simulink model "SignalGen_rx"  (R2016a)
settings: Solver=FixedStepDiscrete  StartTime=0.0  StopTime=0.0333333  RelTol=1e-3
InitFcn:
  | SignalGen_Settings
values from neighbouring files (symbols this model uses):
  A = A(1:L/2+1)    [fft_analisys.m]
  DAC1 = ceil( DAC1_A  * PWM_Counter *             ( DAC1_H1 + DAC1_H2 + DAC1_H3) +               PWM_Offset )    [SignalGen_Pkg_Test.m]    (also in SignalGen_Settings.m)
  DAC2 = ceil( DAC2_A  * PWM_Counter *             ( DAC2_H1 + DAC2_H2 + DAC2_H3 + DAC2_H3) +               PWM_Offset )    [SignalGen_Pkg_Test.m]    (also in SignalGen_Settings.m)
  DAC3 = ceil( DAC3_A  * PWM_Counter *               DAC3_H1 +               PWM_Offset )    [SignalGen_Pkg_Test.m]    (also in SignalGen_Settings.m)
  DAC4 = ceil( DAC4_A  * PWM_Counter *             ( DAC4_H1 + DAC4_noise ) +               PWM_Offset )    [SignalGen_Pkg_Test.m]    (also in SignalGen_Settings.m)
  PWM_Max_Voltage = 3.3    [SignalGen_Pkg_Test.m]    (also in SignalGen_Settings.m)
  PWM_Offset = PWM_Counter/2    (= 180)    [SignalGen_Pkg_Test.m]    (also in SignalGen_Settings.m)
  PWM_Scale = PWM_Max_Voltage/PWM_Counter    (= 0.00916666666667)    [SignalGen_Pkg_Test.m]    (also in SignalGen_Settings.m)
  SampleNumber = 256    [SignalGen_Pkg_Test.m]    (also in SignalGen_Settings.m = 512)
undefined symbols (not defined in the file or in its folder): GPTRIP1SEL, GPTRIP2SEL, TZ1, TZ2
libraries: dspstat3 x4, c2802xlib x2, c280xlib x1, simulink x1
settings Model: ExtModeTrigDuration=8  Creator=Júlio Santos  LastModifiedBy=skelter_win
settings OptimizationCC: DefaultUnderspecifiedDataType=single  OptimizeModelRefInitCode=on  LifeSpan=1  MaxStackSize=512
settings HardwareCC: ProdBitPerChar=16  ProdBitPerInt=16  ProdBitPerPointer=32  ProdLargestAtomicInteger=Integer  ProdLargestAtomicFloat=None  ProdWordSize=16  ProdLongLongMode=on  ProdHWDeviceType=Texas Instruments->C2000
settings RTWCC: SystemTargetFile=ert.tlc  HardwareBoard=TI Piccolo F2806x  TemplateMakefile=ert_default_tmf  GenerateReport=on  Toolchain=Texas Instruments Code Composer Studio v6 (C2000)  BuildConfiguration=Faster Runs  IncludeHyperlinkInReport=on  LaunchReport=on  GenerateTraceInfo=on  GenerateTraceReport=on  GenerateTraceReportSl=on  GenerateTraceReportSf=on  GenerateTraceReportEml=on
settings CodeAppCC: ForceParamTrailComments=on  IgnoreCustomStorageClasses=off  OperatorAnnotations=on  SimulinkDataObjDesc=on  SFDataObjDesc=on  MATLABFcnDesc=on  InsertBlockDesc=on  MATLABSourceComments=on
settings ERTTargetCC: CodeReplacementLibrary=TI C28x  MemSecPackage=Simulink

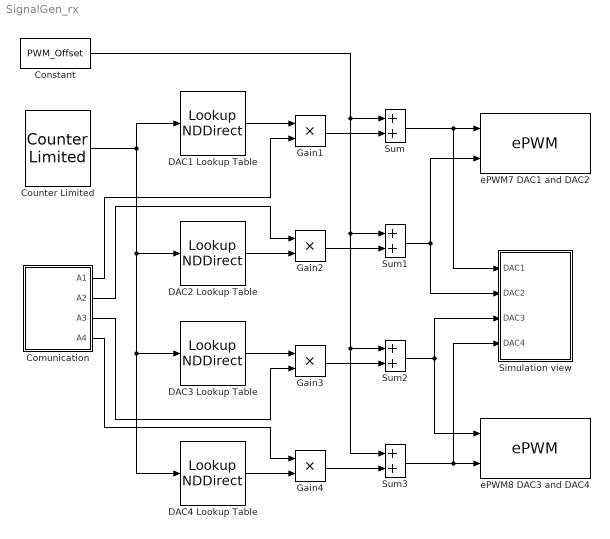
== system SignalGen_rx ==
  Comunication : Subsystem
  Constant : Constant  Value=PWM_Offset
  Counter Limited : simulink/Sources/Counter Limited  uplimit=SampleNumber-1  tsamp=SampleTime
  DAC1 Lookup Table : LookupNDDirect  NumberOfTableDimensions=1  Table=DAC1-PWM_Offset
  DAC2 Lookup Table : LookupNDDirect  NumberOfTableDimensions=1  Table=DAC2-PWM_Offset
  "DAC3 Lookup Table " : LookupNDDirect  NumberOfTableDimensions=1  Table=DAC3-PWM_Offset
  DAC4 Lookup Table : LookupNDDirect  NumberOfTableDimensions=1  Table=DAC4-PWM_Offset
  Gain{1..4} (4 alike) : Product
  Simulation view : Subsystem
  Sum{,1..3} (4 alike) : Sum  OutDataTypeStr=uint16
  ePWM7 DAC1 and DAC2 : c2802xlib/ePWM  useModule=ePWM7  ePWMxLINKTBPRD=Not Linked  periodUnits=Clock cycles  timerSource=Specify via dialog  timerPeriod_clk=PWM_Counter  timerPeriod_sec=2250  tbshadow=Counter equals to zero  countingMode=Up  phaseActiveEnable=Disable  phaseDirection=Count down after sync  phaseActive=0  synchronizationEnable=off  dcaevt1Sync=off  dcbevt1Sync=off  synchronizationOption=Disable  clockPrescale=1  HSclockPrescale=1  enswap=off  ePWMxAStatus=on  ePWMxAactionLogic1=Set  ePWMxAactionLogic2=Clear  ePWMxAactionLogic3=Clear  ePWMxAactionLogic4=Set  ePWMxAactionLogic5=Do nothing  ePWMxAactionLogic6=Do nothing  ePWMxALoadMode=Load on counter equals to zero (CTR=Zero)  ePWMxACSFenable=off  ePWMxACSFvalue=Forcing disable  ePWMxASFreload=Zero  ePWMxBStatus=on  ePWMxBactionLogic1=Set  ePWMxBactionLogic2=Clear  ePWMxBactionLogic3=Do nothing  ePWMxBactionLogic4=Do nothing  ePWMxBactionLogic5=Clear  ePWMxBactionLogic6=Set  ePWMxBLoadMode=Load on counter equals to zero (CTR=Zero)  ePWMxBCSFenable=off  ePWMxBCSFvalue=Forcing disable  ePWMxBSFreload=Zero  ePWNxBOutWay=off  ePWMxLINKCMPA=Not Linked  CMPAUnits=Clock cycles  CMPASource=Input port  CMPAValue_per=50  CMPAValue_clk=PWM_Offset  enCMPAshadow=Counter equals to zero  ePWMxLINKCMPB=Not Linked  CMPBUnits=Clock cycles  CMPBSource=Input port  CMPBValue_per=50  CMPBValue_clk=PWM_Offset  enCMPBshadow=Counter equals to zero  ePWMxLINKCMPC=Not Linked  CMPCUnits=Clock cycles  CMPCSource=Specify via dialog  CMPCValue_per=50  CMPCValue_clk=32000  enCMPCshadow=Counter equals to zero  ePWMxLINKCMPD=Not Linked  CMPDUnits=Clock cycles  CMPDSource=Specify via dialog  CMPDValue_per=50  CMPDValue_clk=32000  enCMPDshadow=Counter equals to zero  enableDBePWMxA=off  enableDBePWMxB=off  enhalfcycle=off  DBpolarity=Active high (AH)  DBedgeDelay=Positive  DBSource_ePWMxA=ePWMxA  DBSource_ePWMxB=ePWMxA  DBperiodSource=Specify via dialog  REDperiod=0  FEDperiod=0  adcstartModuleA=off  adcrequestEventA=First event  adcstartEventA=Digital Compare Module A Event 1 start of conversion (DCAEVT1.soc)  adcstartEventA_type2=Digital Compare Module A Event 1 start of conversion (DCAEVT1.soc)  adcstartModuleB=off  adcrequestEventB=First event  adcstartEventB=Counter equals to zero (CTR=Zero)  adcstartEventB_type2=Counter equals to zero (CTR=Zero)  intEn=off  intPrd=First event  intSel=Counter equals to zero (CTR=Zero)  intSel_type2=Counter equals to zero (CTR=Zero)  hrpe=off  enHRPWM=off  HRPWM_LoadMode=Counter equals to period (CTR=PRD)  HRPWM_CTLMode=Duty or Period control mode  HRPWM_EDGMode=Both edge  hrpeb=off  enHRPWMB=off  HRPWM_LoadModeB=Counter equals to zero (CTR=ZERO)  HRPWM_CTLModeB=Duty or Period control mode  HRPWM_EDGModeB=Both edge  enSFO=on  enautoconv=on  chopperEnable=off  chopperFrequency=1  chopperFirstwidth=1  chopperDuty=12.5%  tripZonesource=Specify via dialog  tzselOSHT1=off  tzselOSHT2=off  tzselOSHT3=off  tzselOSHDCAEV1=off  tzselOSHDCBEV1=off  tzselCBC1=off  tzselCBC2=off  tzselCBC3=off  tzselCBCDCAEV2=off  tzselCBCDCBEV2=off  tzselOSHT4=off  tzselOSHT5=off  tzselOSHT6=off  tzselCBC4=off  tzselCBC5=off  tzselCBC6=off  enTzOstIntr=off  enTzCbcIntr=off  enTzDCAEVT1Intr=off  enTzDCAEVT2Intr=off  enTzDCBEVT1Intr=off  enTzDCBEVT2Intr=off  ePWMxAforced=No action  ePWMxBforced=No action  DCAEVT1forced=No action  DCBEVT1forced=No action  DCAEVT2forced=No action  DCBEVT2forced=No action  dcah=Trip Zone 1 input (TZ1)  dcal=Trip Zone 2 input (TZ2)  dcbh=Trip Zone 1 input (TZ1)  dcbl=Trip Zone 2 input (TZ2)  dcah_type2=GPTRIP1SEL/(TZ1)  dcal_type2=GPTRIP2SEL/(TZ2)  dcbh_type2=GPTRIP1SEL/(TZ1)  dcbl_type2=GPTRIP2SEL/(TZ2)  gendcaevt1=Event disabled  gendcaevt2=Event disabled  gendcbevt1=Event disabled  gendcbevt2=Event disabled  dcaevt1src=DCAEVT1 with sync  dcaevt2src=DCAEVT2 with sync  dcbevt1src=DCBEVT1 with sync  dcbevt2src=DCBEVT2 with sync  pulsesel=Counter equals to zero (CTR=Zero)  blankinv=off  blankoffset=0  blankwidth=0  evsrcsel=Filtered version of DCAEVT1 (DCAEVT1FILT)  encape=off  PwmType=C2000
  ePWM8 DAC3 and DAC4 : c2802xlib/ePWM  useModule=ePWM8  ePWMxLINKTBPRD=Not Linked  periodUnits=Clock cycles  timerSource=Specify via dialog  timerPeriod_clk=PWM_Counter  timerPeriod_sec=2250  tbshadow=Counter equals to zero  countingMode=Up  phaseActiveEnable=Disable  phaseDirection=Count down after sync  phaseActive=0  synchronizationEnable=off  dcaevt1Sync=off  dcbevt1Sync=off  synchronizationOption=Disable  clockPrescale=1  HSclockPrescale=1  enswap=off  ePWMxAStatus=on  ePWMxAactionLogic1=Set  ePWMxAactionLogic2=Clear  ePWMxAactionLogic3=Clear  ePWMxAactionLogic4=Set  ePWMxAactionLogic5=Do nothing  ePWMxAactionLogic6=Do nothing  ePWMxALoadMode=Load on counter equals to zero (CTR=Zero)  ePWMxACSFenable=off  ePWMxACSFvalue=Forcing disable  ePWMxASFreload=Zero  ePWMxBStatus=on  ePWMxBactionLogic1=Set  ePWMxBactionLogic2=Clear  ePWMxBactionLogic3=Do nothing  ePWMxBactionLogic4=Do nothing  ePWMxBactionLogic5=Clear  ePWMxBactionLogic6=Set  ePWMxBLoadMode=Load on counter equals to zero (CTR=Zero)  ePWMxBCSFenable=off  ePWMxBCSFvalue=Forcing disable  ePWMxBSFreload=Zero  ePWNxBOutWay=off  ePWMxLINKCMPA=Not Linked  CMPAUnits=Clock cycles  CMPASource=Input port  CMPAValue_per=50  CMPAValue_clk=PWM_Offset  enCMPAshadow=Counter equals to zero  ePWMxLINKCMPB=Not Linked  CMPBUnits=Clock cycles  CMPBSource=Input port  CMPBValue_per=50  CMPBValue_clk=PWM_Offset  enCMPBshadow=Counter equals to zero  ePWMxLINKCMPC=Not Linked  CMPCUnits=Clock cycles  CMPCSource=Specify via dialog  CMPCValue_per=50  CMPCValue_clk=32000  enCMPCshadow=Counter equals to zero  ePWMxLINKCMPD=Not Linked  CMPDUnits=Clock cycles  CMPDSource=Specify via dialog  CMPDValue_per=50  CMPDValue_clk=32000  enCMPDshadow=Counter equals to zero  enableDBePWMxA=off  enableDBePWMxB=off  enhalfcycle=off  DBpolarity=Active high (AH)  DBedgeDelay=Positive  DBSource_ePWMxA=ePWMxA  DBSource_ePWMxB=ePWMxA  DBperiodSource=Specify via dialog  REDperiod=0  FEDperiod=0  adcstartModuleA=off  adcrequestEventA=First event  adcstartEventA=Digital Compare Module A Event 1 start of conversion (DCAEVT1.soc)  adcstartEventA_type2=Digital Compare Module A Event 1 start of conversion (DCAEVT1.soc)  adcstartModuleB=off  adcrequestEventB=First event  adcstartEventB=Counter equals to zero (CTR=Zero)  adcstartEventB_type2=Counter equals to zero (CTR=Zero)  intEn=off  intPrd=First event  intSel=Counter equals to zero (CTR=Zero)  intSel_type2=Counter equals to zero (CTR=Zero)  hrpe=off  enHRPWM=off  HRPWM_LoadMode=Counter equals to period (CTR=PRD)  HRPWM_CTLMode=Duty or Period control mode  HRPWM_EDGMode=Both edge  hrpeb=off  enHRPWMB=off  HRPWM_LoadModeB=Counter equals to zero (CTR=ZERO)  HRPWM_CTLModeB=Duty or Period control mode  HRPWM_EDGModeB=Both edge  enSFO=on  enautoconv=on  chopperEnable=off  chopperFrequency=1  chopperFirstwidth=1  chopperDuty=12.5%  tripZonesource=Specify via dialog  tzselOSHT1=off  tzselOSHT2=off  tzselOSHT3=off  tzselOSHDCAEV1=off  tzselOSHDCBEV1=off  tzselCBC1=off  tzselCBC2=off  tzselCBC3=off  tzselCBCDCAEV2=off  tzselCBCDCBEV2=off  tzselOSHT4=off  tzselOSHT5=off  tzselOSHT6=off  tzselCBC4=off  tzselCBC5=off  tzselCBC6=off  enTzOstIntr=off  enTzCbcIntr=off  enTzDCAEVT1Intr=off  enTzDCAEVT2Intr=off  enTzDCBEVT1Intr=off  enTzDCBEVT2Intr=off  ePWMxAforced=No action  ePWMxBforced=No action  DCAEVT1forced=No action  DCBEVT1forced=No action  DCAEVT2forced=No action  DCBEVT2forced=No action  dcah=Trip Zone 1 input (TZ1)  dcal=Trip Zone 2 input (TZ2)  dcbh=Trip Zone 1 input (TZ1)  dcbl=Trip Zone 2 input (TZ2)  dcah_type2=GPTRIP1SEL/(TZ1)  dcal_type2=GPTRIP2SEL/(TZ2)  dcbh_type2=GPTRIP1SEL/(TZ1)  dcbl_type2=GPTRIP2SEL/(TZ2)  gendcaevt1=Event disabled  gendcaevt2=Event disabled  gendcbevt1=Event disabled  gendcbevt2=Event disabled  dcaevt1src=DCAEVT1 with sync  dcaevt2src=DCAEVT2 with sync  dcbevt1src=DCBEVT1 with sync  dcbevt2src=DCBEVT2 with sync  pulsesel=Counter equals to zero (CTR=Zero)  blankinv=off  blankoffset=0  blankwidth=0  evsrcsel=Filtered version of DCAEVT1 (DCAEVT1FILT)  encape=off  PwmType=C2000
  wires:
  Counter Limited/1 -> DAC1 Lookup Table/1, DAC4 Lookup Table/1, "DAC3 Lookup Table "/1, DAC2 Lookup Table/1
  DAC2 Lookup Table/1 -> Gain2/2
  Gain1/1 -> Sum/2
  Gain2/1 -> Sum1/2
  DAC4 Lookup Table/1 -> Gain4/2
  Sum/1 -> Simulation view/1(DAC1), ePWM7 DAC1 and DAC2/1
  Constant/1 -> Sum3/1, Sum2/1, Sum1/1, Sum/1
  Sum1/1 -> ePWM7 DAC1 and DAC2/2, Simulation view/2(DAC2)
  Gain3/1 -> Sum2/2
  Gain4/1 -> Sum3/2
  Sum2/1 -> ePWM8 DAC3 and DAC4/1, Simulation view/3(DAC3)
  Sum3/1 -> Simulation view/4(DAC4), ePWM8 DAC3 and DAC4/2
  Comunication/1(A1) -> Gain1/2
  DAC1 Lookup Table/1 -> Gain1/1
  Comunication/2(A2) -> Gain2/1
  Comunication/4(A4) -> Gain4/1
  "DAC3 Lookup Table "/1 -> Gain3/1
  Comunication/3(A3) -> Gain3/2

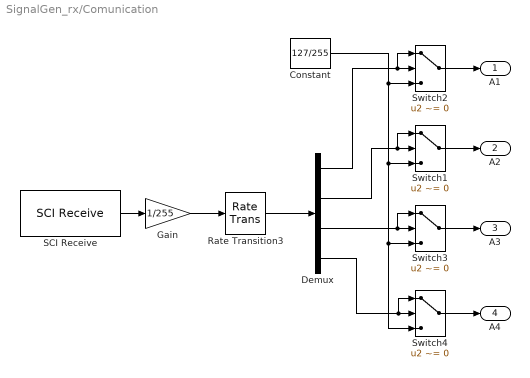
== system SignalGen_rx/Comunication ==
  Constant : Constant  Value=127/255
  Demux : Demux
  Gain : Gain  Gain=1/255
  Rate Transition3 : RateTransition  Integrity=off
  SCI Receive : c280xlib/SCI Receive  sciModule=A  dataHead='S'  dataTail='E'  dataType=uint8  dataDim=4  initValue=0  errOption=Output the last received value  errValue=0  sampleTime=0.05  outputStatus=off  postInterrupt=off  numFifo=1
  Switch{1..4} (4 alike) : Switch  Criteria=u2 ~= 0
  A1 : Outport
  A2 : Outport  Port=2
  A3 : Outport  Port=3
  A4 : Outport  Port=4
  wires:
  SCI Receive/1 -> Gain/1
  Gain/1 -> Rate Transition3/1
  Rate Transition3/1 -> Demux/1
  Demux/1 -> Switch2/1, Switch2/2
  Switch2/1 -> A1/1
  Constant/1 -> Switch2/3, Switch1/3, Switch4/3, Switch3/3
  Switch1/1 -> A2/1
  Demux/2 -> Switch1/1, Switch1/2
  Switch3/1 -> A3/1
  Demux/3 -> Switch3/1, Switch3/2
  Switch4/1 -> A4/1
  Demux/4 -> Switch4/1, Switch4/2

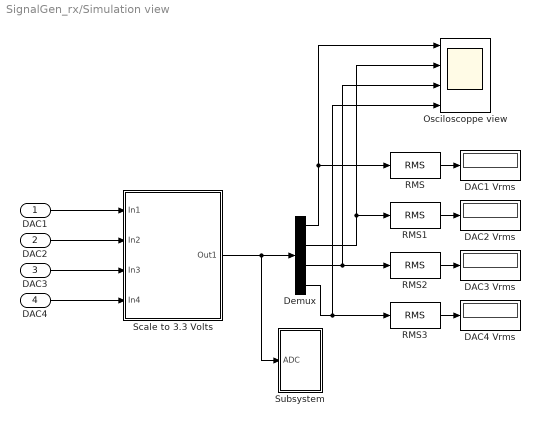
== system SignalGen_rx/Simulation view ==
  DAC1 : Inport
  DAC2 : Inport  Port=2
  DAC3 : Inport  Port=3
  DAC4 : Inport  Port=4
  DAC1 Vrms : Display
  DAC2 Vrms : Display
  DAC3 Vrms : Display
  DAC4 Vrms : Display
  Demux : Demux
  Osciloscoppe view : Scope  NumInputPorts=4
  RMS{,1..3} (4 alike) : dspstat3/RMS  run=on  reset_popup=None  InputProcessing=Columns as channels (frame based)  directionMode=Each column  dimension=1
  Scale to 3.3 Volts : Subsystem
  Subsystem : Subsystem
  wires:
  RMS1/1 -> DAC2 Vrms/1
  RMS2/1 -> DAC3 Vrms/1
  RMS3/1 -> DAC4 Vrms/1
  RMS/1 -> DAC1 Vrms/1
  Demux/1 -> Osciloscoppe view/1, RMS/1
  Demux/4 -> Osciloscoppe view/4, RMS3/1
  Demux/2 -> Osciloscoppe view/2, RMS1/1
  Demux/3 -> Osciloscoppe view/3, RMS2/1
  Scale to 3.3 Volts/1(Out1) -> Subsystem/1(ADC), Demux/1
  DAC1/1 -> Scale to 3.3 Volts/1(In1)
  DAC2/1 -> Scale to 3.3 Volts/2(In2)
  DAC3/1 -> Scale to 3.3 Volts/3(In3)
  DAC4/1 -> Scale to 3.3 Volts/4(In4)

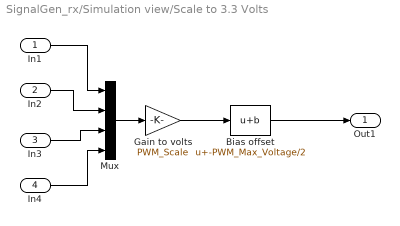
== system SignalGen_rx/Simulation view/Scale to 3.3 Volts ==
  In1 : Inport
  In2 : Inport  Port=2
  In3 : Inport  Port=3
  In4 : Inport  Port=4
  Bias offset : Bias  Bias=-PWM_Max_Voltage/2
  Gain to volts : Gain  Gain=PWM_Scale  OutDataTypeStr=single
  Mux : Mux
  Out1 : Outport
  wires:
  In1/1 -> Mux/1
  In4/1 -> Mux/4
  In3/1 -> Mux/3
  In2/1 -> Mux/2
  Bias offset/1 -> Out1/1
  Gain to volts/1 -> Bias offset/1
  Mux/1 -> Gain to volts/1

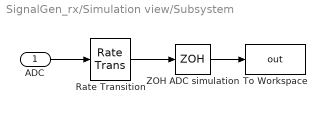
== system SignalGen_rx/Simulation view/Subsystem ==
  ADC : Inport
  Rate Transition : RateTransition  Integrity=off
  To Workspace : ToWorkspace  VariableName=out  SaveFormat=Structure With Time  SampleTime=-1
  ZOH ADC simulation : ZeroOrderHold  SampleTime=1/(60*256)
  wires:
  ZOH ADC simulation/1 -> To Workspace/1
  Rate Transition/1 -> ZOH ADC simulation/1
  ADC/1 -> Rate Transition/1
